simulink model "inverter_fault_mc_sim"  (R2016a)
settings: Solver=ode4  StartTime=0.0  StopTime=Tfinal  FixedStep=Ts  RelTol=1e-3
values from neighbouring files (symbols this model uses):
  Cdc = 200e-6    (= 0.0002)    [inverter_fault_sim.m]
  delta = acos(Ef/Vt)    [inverter_fault_sim.m]
  Foct = 0    [inverter_fault_sim.m]
  Focw = 1    [inverter_fault_sim.m]
  Fs = 0.0005    [inverter_fault_sim.m]
  Fsct = 0    [inverter_fault_sim.m]
  Fscw = 0    [inverter_fault_sim.m]
  Jm = 0.003    [inverter_fault_sim.m]
  ma = Vt*sqrt(3)/(Vdcm*0.612)    [inverter_fault_sim.m]
  Nr = 600    [inverter_fault_sim.m]    (also in short_circuit.m)
  p = 10    [fault_tolerance_torque.m]    (also in inverter_fault_sim.m; short_circuit.m = 20)
  phase = 0*pi/180    (= 0)    [fault_tolerance_torque.m]    (also in inverter_fault_sim.m = [0 90 0 90])
  Rin = 10    [inverter_fault_sim.m]
  Ripth = 0.15    [inverter_fault_sim.m]
  Roc = 1e4    (= 10000)    [inverter_fault_sim.m]
  Rs = 0.277e-6    (= 2.77e-07)    [inverter_fault_sim.m]    (also in short_circuit.m = 0.277)
  Tfault = 0    [inverter_fault_sim.m]
  Tm = Tma + Tmb + Tmc    [fault_tolerance_torque.m]    (also in inverter_fault_sim.m = 127)
  Ts = 1e-6    (= 1e-06)    [inverter_fault_sim.m]
  Vin = Vdc + Rin*(Pout/Vdc)    (= 675.030864198)    [inverter_fault_sim.m]
  wout = 2*pi*fout    (= 628.318530718)    [inverter_fault_sim.m]
undefined symbols (not defined in the file or in its folder): Lload, Rload
libraries: powerlib x32, powerlib_meascontrol x7, simulink x2
settings Model: Creator=ugurm  LastModifiedBy=mesutto
settings DataIOCC: LimitDataPoints=on  SaveFormat=Array
settings DebuggingCC: UnderspecifiedInitializationDetection=Classic  MergeDetectMultiDrivingBlocksExec=none  SolverPrmCheckMsg=warning  StateNameClashWarn=warning
settings HardwareCC: ProdBitPerPointer=32  ProdLargestAtomicFloat=None  ProdIntDivRoundTo=Undefined  ProdEndianess=Unspecified  ProdWordSize=32  ProdHWDeviceType=32-bit Generic
settings ModelReferenceCC: PropagateSignalLabelsOutOfModel=off
settings ConfigComp: CovModelRefEnable=Off

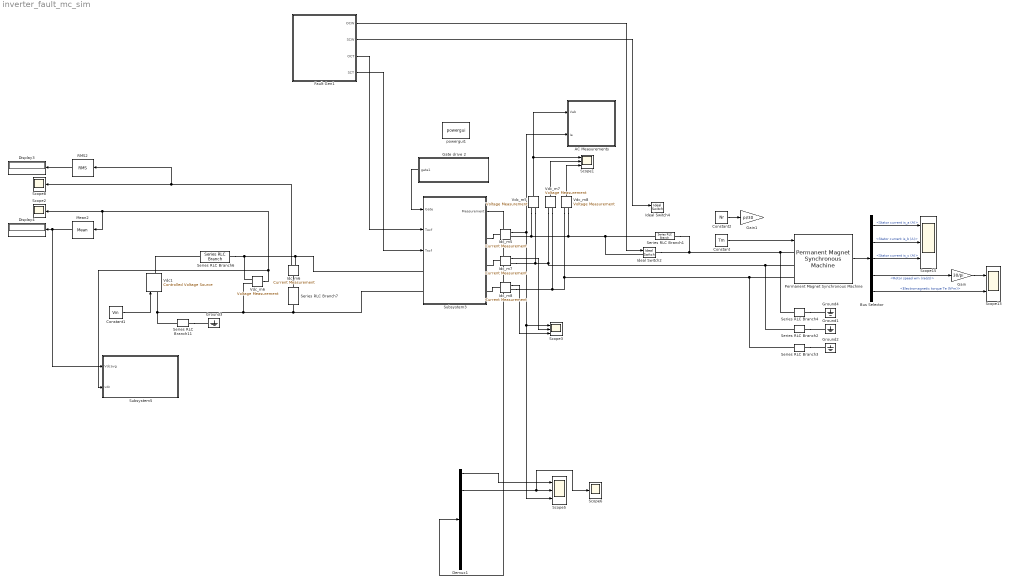
== system inverter_fault_mc_sim ==
  AC Measurements : Subsystem
  Bus Selector : BusSelector  OutputSignals=Stator current is_a (A),Stator current is_b (A),Stator current is_c (A),Rotor speed wm (rad/s),Electromagnetic torque Te (N*m)
  Constant : Constant  Value=Tm
  Constant1 : Constant  Value=Vin
  Constant2 : Constant  Value=Nr
  Demux1 : Demux  Outputs=12
  Display3 : Display
  Display4 : Display
  Fault Gen1 : Subsystem
  Gain : Gain  Gain=30/pi
  Gain1 : Gain  Gain=pi/30
  Gate drive 2 : Subsystem
  Ground{1..4} (4 alike) : powerlib/Elements/Ground  LConnTagsString=a
  Idc_m{5..8} (4 alike) : powerlib/Measurements/Current Measurement  PhasorSimulation=off  OutputType=Complex  PSBequivalent=0
  Ideal Switch2 : powerlib/Power Electronics/Ideal Switch  Ron=0.001  Lon=0  IC=0  Rs=1e9  Cs=inf  Measurements=off
  Ideal Switch4 : powerlib/Power Electronics/Ideal Switch  Ron=0.001  Lon=0  IC=0  Rs=1e9  Cs=inf  Measurements=off
  Mean2 : powerlib_meascontrol/Measurements/Mean  Freq=fout  Vinit=0  Ts=0
  Permanent Magnet Synchronous Machine : powerlib/Machines/Permanent Magnet Synchronous Machine  NbPhases=3  FluxDistribution=Sinusoidal  RotorType=Round  MechanicalLoad=Torque Tm  PresetModel=No  ShowDetailedParameters=on  MeasurementBus=off  Resistance=Rs  Inductance=8.5e-3  dqInductances=[8.5e-3,8.5e-3]  La=Ls  MachineConstant=Voltage Constant (V_peak L-L / krpm)  Flux=0.36013  VoltageCst=Vcon  TorqueCst=5.4019  Flat=120  Mechanical=[Jm Fs p 0]  PolePairs=4  InitialConditions=[0,0, 0,0]  InitialConditions5ph=[0 0 0 0 0 0]  TsPowergui=0  TsBlock=-1  RefAngle=90 degrees behind phase A axis (modified Park)
      link override From: GotoTag=T63_6243_6509680743507
  RMS2 : powerlib_meascontrol/Measurements/RMS  TrueRMS=on  Freq=fout  RMSInit=0  Ts=0
  Scope{1,3,5,15} (4 alike) : Scope  NumInputPorts=3
  Scope13 : Scope  NumInputPorts=2
  Scope2 : Scope
  Scope6 : Scope
  Scope8 : Scope
  Series RLC Branch1 : powerlib/Elements/Series RLC Branch  LConnTagsString=__new0  RConnTagsString=__new0  BranchType=R  Resistance=Roc  Inductance=Lload  SetiL0=off  InitialCurrent=0  Capacitance=1e-6  Setx0=off  InitialVoltage=0  Measurements=None
  Series RLC Branch{2..4,11} (4 alike) : powerlib/Elements/Series RLC Branch  LConnTagsString=__new0  RConnTagsString=__new0  BranchType=R  Resistance=1e12  Inductance=Lload  SetiL0=off  InitialCurrent=0  Capacitance=1e-6  Setx0=off  InitialVoltage=0  Measurements=None
  Series RLC Branch6 : powerlib/Elements/Series RLC Branch  LConnTagsString=__new0  RConnTagsString=__new0  BranchType=R  Resistance=Rin  Inductance=Lload  SetiL0=off  InitialCurrent=0  Capacitance=1e-6  Setx0=off  InitialVoltage=0  Measurements=None
  Series RLC Branch7 : powerlib/Elements/Series RLC Branch  LConnTagsString=__new0  RConnTagsString=__new0  BranchType=C  Resistance=Rload  Inductance=Lload  SetiL0=off  InitialCurrent=0  Capacitance=Cdc  Setx0=off  InitialVoltage=0  Measurements=None
  Subsystem3 : Subsystem
  Subsystem5 : Subsystem
  Vdc1 : powerlib/Electrical Sources/Controlled Voltage Source  Initialize=off  Source_Type=DC  Amplitude=200  Phase=0  Frequency=0  Measurements=None
  Vdc_m{5..8} (4 alike) : powerlib/Measurements/Voltage Measurement  PhasorSimulation=off  OutputType=Complex  PSBequivalent=0
  powergui1 : powerlib/powergui  Priority=1  SimulationMode=Discrete  SolverType=Tustin  SampleTime=Ts  frequency=60  SPID=off  DisableSnubberDevices=off  DisableRonSwitches=off  DisableVfSwitches=off  SwTol=0  DisplayEquations=off  Interpol=off  ExternalGateDelay=off  methode=off  Ts=0  FunctionMessages=off  echomessages=off  HookPort=off  EnableUseOfTLC=off  x0status=blocks  frequencyindice=0  Pbase=100e6  ErrMax=1e-4  Iterations=50  UnitsV=kV  UnitsW=MW  buscounter=0  RestoreLinks=warning  ResistiveCurrentMeasurement=off  Frange=[0:2:500]  Ylog=off  Xlog=on  ShowGrid=off  save=off  variable=ZData  structure=Vdc  ZoomFFT=off  StartTime=0.04  cycles=5  DisplayStyle=5  fundamental=50  FreqAxis=off  MaxFrequency=30000  frequencyindicesteady=1  RmsSteady=1  display=off
  wires:
  Gate drive 2/1(gate1) -> Subsystem3/1(Gate)
  Vdc_m5/1 -> AC Measurements/1(Vab), Scope1/1
  Idc_m5/1 -> AC Measurements/2(Ia), Scope5/3, Scope3/1
  Constant1/1 -> Vdc1/1
  Idc_m6/1 -> RMS2/1, Scope8/1
  Vdc_m6/1 -> Subsystem5/2(vdc), Mean2/1, Scope2/1
  Idc_m7/1 -> Scope3/2
  Idc_m8/1 -> Scope3/3
  RMS2/1 -> Display3/1
  Vdc_m7/1 -> Scope1/2
  Vdc_m8/1 -> Scope1/3
  Mean2/1 -> Subsystem5/1(Vdcavg), Display4/1
  Demux1/1 -> Scope5/1
  Demux1/3 -> Scope6/1, Scope5/2
  Subsystem3/1(Measurement) -> Demux1/1
  Fault Gen1/4(SCT) -> Subsystem3/3(Tscf)
  Fault Gen1/3(OCT) -> Subsystem3/2(Tocf)
  Fault Gen1/2(SCW) -> Ideal Switch4/1
  Fault Gen1/1(OCW) -> Ideal Switch2/1
  Permanent Magnet Synchronous Machine/1 -> Bus Selector/1
  Bus Selector/1 -> Scope15/1  "<Stator current is_a (A)>"
  Bus Selector/2 -> Scope15/2  "<Stator current is_b (A)>"
  Bus Selector/3 -> Scope15/3  "<Stator current is_c (A)>"
  Bus Selector/4 -> Gain/1  "<Rotor speed wm (rad/s)>"
  Bus Selector/5 -> Scope13/2  "<Electromagnetic torque Te (N*m)>"
  Gain/1 -> Scope13/1
  Constant2/1 -> Gain1/1
  Constant/1 -> Permanent Magnet Synchronous Machine/1
  connections:
  Series RLC Branch1/RConn1 -- Ideal Switch2/RConn1 -- Series RLC Branch4/LConn1 -- Permanent Magnet Synchronous Machine/LConn1
  Vdc1/LConn1 -- Series RLC Branch11/LConn1 -- Vdc_m6/LConn2 -- Series RLC Branch7/RConn1 -- Subsystem3/LConn2
  Idc_m6/RConn1 -- Subsystem3/LConn1 -- Series RLC Branch6/RConn1 -- Vdc_m6/LConn1
  Vdc_m7/LConn2 -- Series RLC Branch3/LConn1 -- Permanent Magnet Synchronous Machine/LConn3 -- Vdc_m8/LConn1 -- Idc_m8/RConn1
  Vdc_m7/LConn1 -- Series RLC Branch2/LConn1 -- Permanent Magnet Synchronous Machine/LConn2 -- Vdc_m5/LConn2 -- Idc_m7/RConn1
  Vdc1/RConn1 -- Series RLC Branch6/LConn1
  Idc_m6/LConn1 -- Series RLC Branch7/LConn1
  Idc_m8/LConn1 -- Subsystem3/RConn3
  Series RLC Branch11/RConn1 -- Ground3/LConn1
  Subsystem3/RConn1 -- Idc_m5/LConn1
  Idc_m7/LConn1 -- Subsystem3/RConn2
  Vdc_m8/LConn2 -- Ideal Switch2/LConn1 -- Series RLC Branch1/LConn1 -- Idc_m5/RConn1 -- Vdc_m5/LConn1
  Series RLC Branch2/RConn1 -- Ground1/LConn1
  Series RLC Branch3/RConn1 -- Ground2/LConn1
  Series RLC Branch4/RConn1 -- Ground4/LConn1

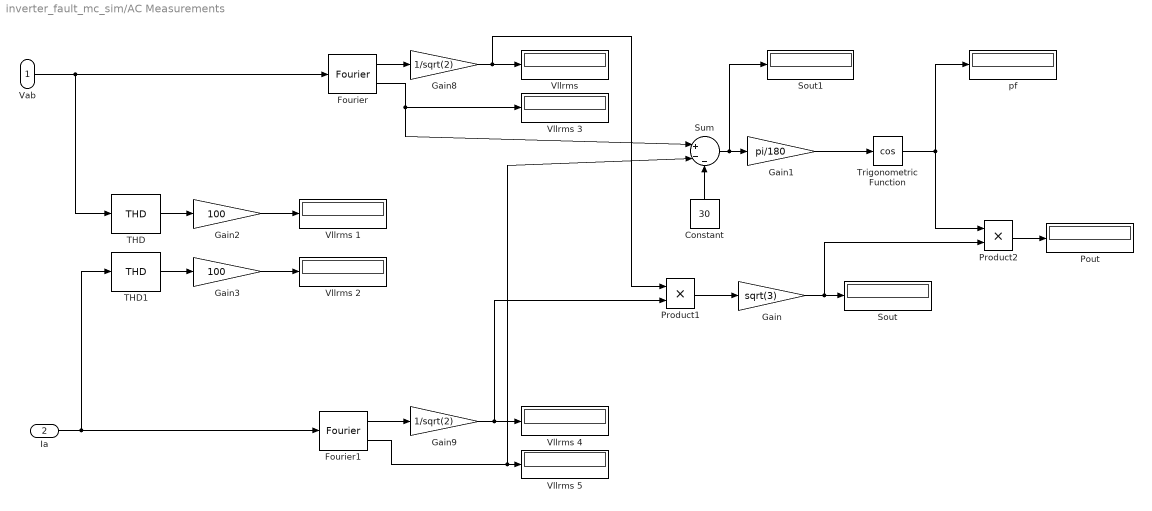
== system inverter_fault_mc_sim/AC Measurements ==
  Vab : Inport
  Ia : Inport  Port=2
  Constant : Constant  Value=30
  Fourier : powerlib_meascontrol/Measurements/Fourier  Freq=fout  n=1  InInit=[0, 0]  Ts=Ts
  Fourier1 : powerlib_meascontrol/Measurements/Fourier  Freq=fout  n=1  InInit=[0, 0]  Ts=Ts
  Gain : Gain  Gain=sqrt(3)
  Gain1 : Gain  Gain=pi/180
  Gain2 : Gain  Gain=100
  Gain3 : Gain  Gain=100
  Gain8 : Gain  Gain=1/sqrt(2)
  Gain9 : Gain  Gain=1/sqrt(2)
  Pout : Display
  Product1 : Product
  Product2 : Product
  Sout : Display
      settings: Format=short_e
  Sout1 : Display
      settings: Format=short_e
  Sum : Sum  Inputs=|+--
  THD : powerlib_meascontrol/Measurements/THD  Freq=fout  Ts=0
  THD1 : powerlib_meascontrol/Measurements/THD  Freq=fout  Ts=0
  Trigonometric Function : Trigonometry  Operator=cos
  Vllrms {,1..5} (6 alike) : Display
  pf : Display
  wires:
  Gain8/1 -> "Vllrms "/1, Product1/1
  Gain9/1 -> Vllrms 4/1, Product1/2
  Ia/1 -> THD1/1, Fourier1/1
  Fourier1/1 -> Gain9/1
  Vab/1 -> THD/1, Fourier/1
  Fourier/1 -> Gain8/1
  Product1/1 -> Gain/1
  Gain1/1 -> Trigonometric Function/1
  Product2/1 -> Pout/1
  Fourier/2 -> Sum/1, Vllrms 3/1
  THD/1 -> Gain2/1
  THD1/1 -> Gain3/1
  Fourier1/2 -> Sum/2, Vllrms 5/1
  Gain2/1 -> Vllrms 1/1
  Gain3/1 -> Vllrms 2/1
  Gain/1 -> Product2/2, Sout/1
  Sum/1 -> Sout1/1, Gain1/1
  Constant/1 -> Sum/3
  Trigonometric Function/1 -> pf/1, Product2/1

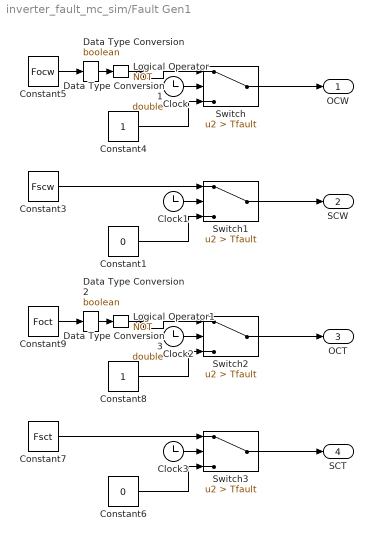
== system inverter_fault_mc_sim/Fault Gen1 ==
  Clock{,1..3} (4 alike) : Clock
  Constant1 : Constant  Value=0
  Constant3 : Constant  Value=Fscw
  Constant4 : Constant
  Constant5 : Constant  Value=Focw
  Constant6 : Constant  Value=0
  Constant7 : Constant  Value=Fsct
  Constant8 : Constant
  Constant9 : Constant  Value=Foct
  Data Type Conversion : DataTypeConversion  OutDataTypeStr=boolean
  Data Type Conversion1 : DataTypeConversion  OutDataTypeStr=double
  Data Type Conversion2 : DataTypeConversion  OutDataTypeStr=boolean
  Data Type Conversion3 : DataTypeConversion  OutDataTypeStr=double
  Logical Operator : Logic  Operator=NOT  AllPortsSameDT=off  OutDataTypeStr=boolean
  Logical Operator1 : Logic  Operator=NOT  AllPortsSameDT=off  OutDataTypeStr=boolean
  Switch{,1..3} (4 alike) : Switch  Criteria=u2 > Threshold  Threshold=Tfault
  OCW : Outport
  SCW : Outport  Port=2
  OCT : Outport  Port=3
  SCT : Outport  Port=4
  wires:
  Data Type Conversion1/1 -> Switch/1
  Data Type Conversion/1 -> Logical Operator/1
  Logical Operator/1 -> Data Type Conversion1/1
  Constant5/1 -> Data Type Conversion/1
  Constant1/1 -> Switch1/3
  Constant3/1 -> Switch1/1
  Clock1/1 -> Switch1/2
  Switch1/1 -> SCW/1
  Switch/1 -> OCW/1
  Constant4/1 -> Switch/3
  Clock/1 -> Switch/2
  Clock2/1 -> Switch2/2
  Clock3/1 -> Switch3/2
  Constant6/1 -> Switch3/3
  Switch2/1 -> OCT/1
  Data Type Conversion3/1 -> Switch2/1
  Constant9/1 -> Data Type Conversion2/1
  Constant8/1 -> Switch2/3
  Logical Operator1/1 -> Data Type Conversion3/1
  Data Type Conversion2/1 -> Logical Operator1/1
  Constant7/1 -> Switch3/1
  Switch3/1 -> SCT/1

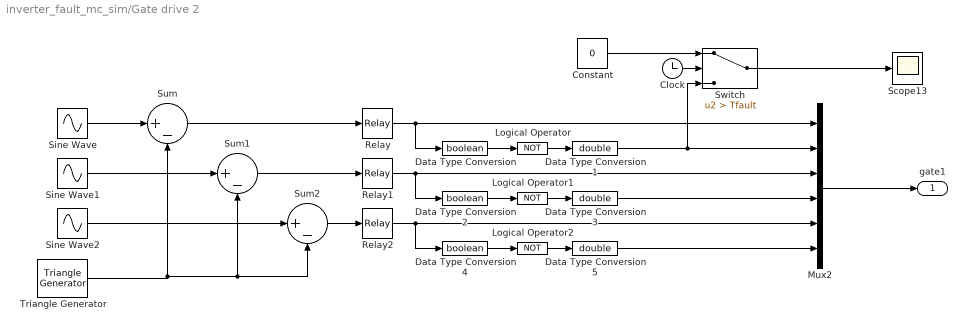
== system inverter_fault_mc_sim/Gate drive 2 ==
  Clock : Clock
  Constant : Constant  Value=0
  Data Type Conversion : DataTypeConversion  OutDataTypeStr=boolean
  Data Type Conversion1 : DataTypeConversion  OutDataTypeStr=double
  Data Type Conversion2 : DataTypeConversion  OutDataTypeStr=boolean
  Data Type Conversion3 : DataTypeConversion  OutDataTypeStr=double
  Data Type Conversion4 : DataTypeConversion  OutDataTypeStr=boolean
  Data Type Conversion5 : DataTypeConversion  OutDataTypeStr=double
  Logical Operator : Logic  Operator=NOT  AllPortsSameDT=off  OutDataTypeStr=boolean
  Logical Operator1 : Logic  Operator=NOT  AllPortsSameDT=off  OutDataTypeStr=boolean
  Logical Operator2 : Logic  Operator=NOT  AllPortsSameDT=off  OutDataTypeStr=boolean
  Mux2 : Mux  Inputs=6
  Relay : Relay
  Relay1 : Relay
  Relay2 : Relay
  Scope13 : Scope
  Sine Wave : Sin  Amplitude=ma  Frequency=wout  Phase=delta  SampleTime=0
  Sine Wave1 : Sin  Amplitude=ma  Frequency=wout  Phase=-2*pi/3+delta  SampleTime=0
  Sine Wave2 : Sin  Amplitude=ma  Frequency=wout  Phase=2*pi/3+delta  SampleTime=0
  Sum : Sum  Inputs=|+-
  Sum1 : Sum  Inputs=|+-
  Sum2 : Sum  Inputs=|+-
  Switch : Switch  Criteria=u2 > Threshold  Threshold=Tfault
  Triangle Generator : powerlib_meascontrol/Pulse & Signal Generators/Triangle Generator  Freq=fsw  Phase=phase(1)  Ts=Ts
  gate1 : Outport
  wires:
  Sine Wave/1 -> Sum/1
  Triangle Generator/1 -> Sum1/2, Sum2/2, Sum/2
  Sine Wave1/1 -> Sum1/1
  Sine Wave2/1 -> Sum2/1
  Sum/1 -> Relay/1
  Sum1/1 -> Relay1/1
  Sum2/1 -> Relay2/1
  Data Type Conversion/1 -> Logical Operator/1
  Relay/1 -> Data Type Conversion/1, Mux2/1
  Logical Operator/1 -> Data Type Conversion1/1
  Data Type Conversion2/1 -> Logical Operator1/1
  Relay1/1 -> Data Type Conversion2/1, Mux2/3
  Logical Operator1/1 -> Data Type Conversion3/1
  Data Type Conversion3/1 -> Mux2/4
  Data Type Conversion4/1 -> Logical Operator2/1
  Relay2/1 -> Data Type Conversion4/1, Mux2/5
  Logical Operator2/1 -> Data Type Conversion5/1
  Data Type Conversion5/1 -> Mux2/6
  Mux2/1 -> gate1/1
  Clock/1 -> Switch/2
  Switch/1 -> Scope13/1
  Constant/1 -> Switch/1
  Data Type Conversion1/1 -> Mux2/2, Switch/3

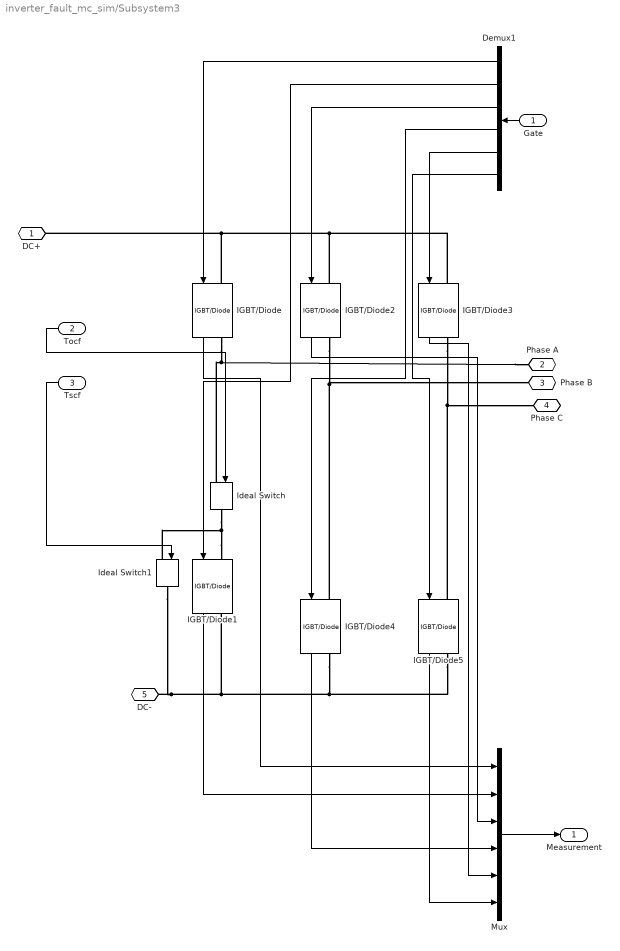
== system inverter_fault_mc_sim/Subsystem3 ==
  Gate : Inport
  Tocf : Inport  Port=2
  Tscf : Inport  Port=3
  Demux1 : Demux  Outputs=6
  IGBT/Diode{,1..5} (6 alike) : powerlib/Power Electronics/IGBT//Diode  Ron=1e-3  Rs=1e5  Cs=inf  Measurements=on
  Ideal Switch : powerlib/Power Electronics/Ideal Switch  Ron=0.001  Lon=0  IC=0  Rs=inf  Cs=inf  Measurements=off
  Ideal Switch1 : powerlib/Power Electronics/Ideal Switch  Ron=0.001  Lon=0  IC=0  Rs=inf  Cs=inf  Measurements=off
  Mux : Mux  Inputs=6
  DC+ : PMIOPort  Port=1  Side=Left
  Phase A : PMIOPort  Port=2  Side=Right
  Phase B : PMIOPort  Port=3  Side=Right
  Phase C : PMIOPort  Port=4  Side=Right
  DC- : PMIOPort  Port=5  Side=Left
  Measurement : Outport
  wires:
  Gate/1 -> Demux1/1
  Demux1/4 -> IGBT/Diode4/1
  Demux1/2 -> IGBT/Diode1/1
  Demux1/3 -> IGBT/Diode2/1
  Demux1/5 -> IGBT/Diode3/1
  Demux1/6 -> IGBT/Diode5/1
  Demux1/1 -> IGBT/Diode/1
  IGBT/Diode/1 -> Mux/1
  IGBT/Diode1/1 -> Mux/2
  IGBT/Diode2/1 -> Mux/3
  IGBT/Diode4/1 -> Mux/4
  IGBT/Diode3/1 -> Mux/5
  IGBT/Diode5/1 -> Mux/6
  Mux/1 -> Measurement/1
  Tocf/1 -> Ideal Switch/1
  Tscf/1 -> Ideal Switch1/1
  connections:
  IGBT/Diode3/RConn1 -- Phase C/RConn1 -- IGBT/Diode5/LConn1
  IGBT/Diode2/LConn1 -- IGBT/Diode/LConn1 -- DC+/RConn1 -- IGBT/Diode3/LConn1
  IGBT/Diode1/RConn1 -- IGBT/Diode5/RConn1 -- IGBT/Diode4/RConn1 -- DC-/RConn1 -- Ideal Switch1/RConn1
  Phase A/RConn1 -- IGBT/Diode/RConn1 -- Ideal Switch/LConn1
  IGBT/Diode2/RConn1 -- Phase B/RConn1 -- IGBT/Diode4/LConn1
  IGBT/Diode1/LConn1 -- Ideal Switch/RConn1 -- Ideal Switch1/LConn1

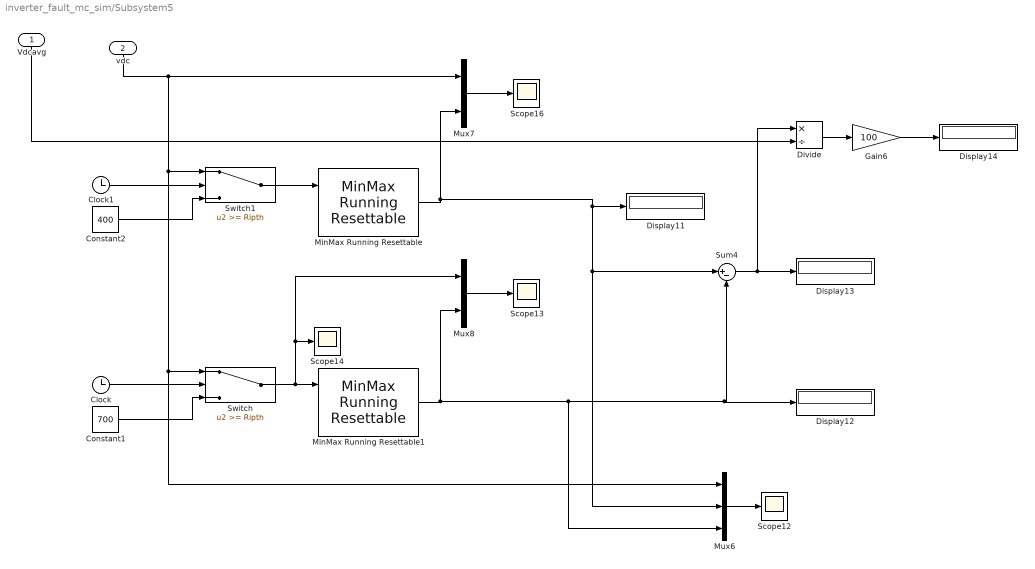
== system inverter_fault_mc_sim/Subsystem5 ==
  Vdcavg : Inport
  vdc : Inport  Port=2
  Clock : Clock
  Clock1 : Clock
  Constant1 : Constant  Value=700  SampleTime=Ts
  Constant2 : Constant  Value=400  SampleTime=Ts
  Display{11..14} (4 alike) : Display
  Divide : Product  Inputs=*/
  Gain6 : Gain  Gain=100
  MinMax Running Resettable : simulink/Math Operations/MinMax Running Resettable  Function=max  vinit=0.0
  MinMax Running Resettable1 : simulink/Math Operations/MinMax Running Resettable  Function=min  vinit=700
  Mux6 : Mux  Inputs=3
  Mux7 : Mux  Inputs=2
  Mux8 : Mux  Inputs=2
  Scope{12..14,16} (4 alike) : Scope
  Sum4 : Sum  Inputs=|+-
  Switch : Switch  Threshold=Ripth
  Switch1 : Switch  Threshold=Ripth
  wires:
  MinMax Running Resettable/1 -> Display11/1, Mux6/2, Sum4/1, Mux7/2
  Clock/1 -> Switch/2
  Mux8/1 -> Scope13/1
  Gain6/1 -> Display14/1
  Constant1/1 -> Switch/3
  MinMax Running Resettable1/1 -> Mux6/3, Display12/1, Sum4/2, Mux8/2
  Mux7/1 -> Scope16/1
  Switch/1 -> Mux8/1, Scope14/1, MinMax Running Resettable1/1
  Sum4/1 -> Divide/1, Display13/1
  Divide/1 -> Gain6/1
  Mux6/1 -> Scope12/1
  Vdcavg/1 -> Divide/2
  vdc/1 -> Mux7/1, Switch1/1, Mux6/1, Switch/1
  Switch1/1 -> MinMax Running Resettable/1
  Clock1/1 -> Switch1/2
  Constant2/1 -> Switch1/3
